simulink model "reservoir"  (R2016a)
settings: Solver=VariableStepAuto  StartTime=0.0  StopTime=10.0  RelTol=1e-3
settings Model: Creator=desilvtk  LastModifiedBy=desilvtk

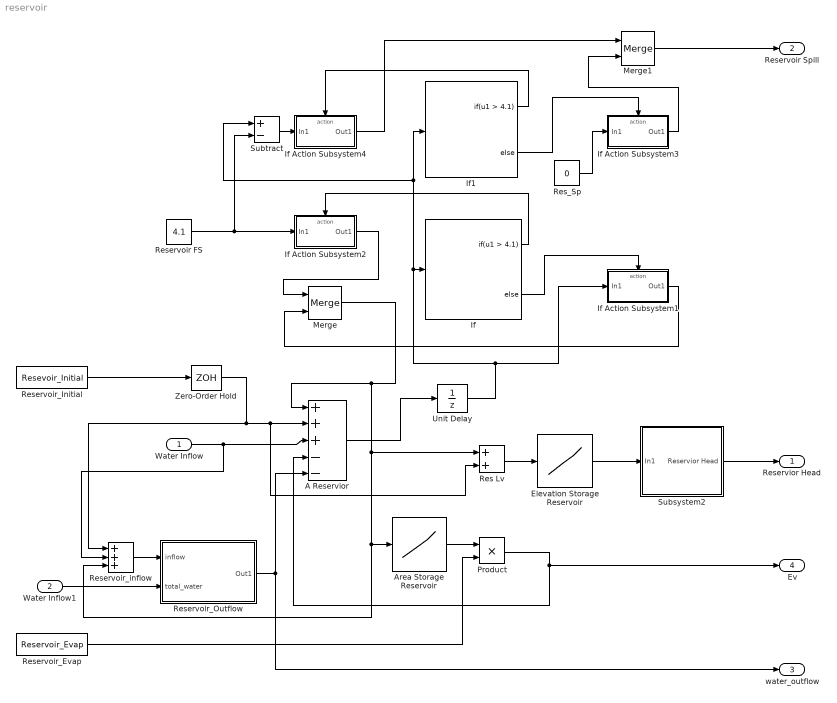
== system reservoir ==
  Water Inflow : Inport
  Water Inflow1 : Inport  Port=2
  A Reservior : Sum  Inputs=+++--
  Area Storage Reservoir : Lookup_n-D  NumberOfTableDimensions=1  BreakpointsForDimension1=[1.7,2.4,3.3,4.1]  UseOneInputPortForAllInputData=on  Table=[0.6,0.8,1,1.2]  InternalRulePriority=Speed  RndMeth=Simplest  InputSameDT=on
  Elevation Storage Reservoir : Lookup_n-D  NumberOfTableDimensions=1  BreakpointsForDimension1=[1.7,2.4,3.3,4.1]  UseOneInputPortForAllInputData=on  Table=[0,1,2,2]  InternalRulePriority=Speed  RndMeth=Simplest  InputSameDT=on
  If : If  IfExpression=u1 > 4.1
  If Action Subsystem1 : Subsystem  TreatAsAtomicUnit=on
  If Action Subsystem2 : Subsystem  TreatAsAtomicUnit=on
  If Action Subsystem3 : Subsystem  TreatAsAtomicUnit=on
  If Action Subsystem4 : Subsystem  TreatAsAtomicUnit=on
  If1 : If  IfExpression=u1 > 4.1
  Merge : Merge
  Merge1 : Merge
  Product : Product
  Res Lv : Sum
  Res_Sp : Constant  Value=0
  Reservoir FS : Constant  Value=4.1
  Reservoir_Evap : FromWorkspace  VariableName=Reservoir_Evap  SampleTime=0
  Reservoir_Initial : FromWorkspace  VariableName=Resevoir_Initial  SampleTime=0
  Reservoir_Outflow : Subsystem
  Reservoir_inflow : Sum  Inputs=+++
  Subsystem2 : Subsystem
  Subtract : Sum  Inputs=+-
  Unit Delay : UnitDelay
  Zero-Order Hold : ZeroOrderHold
  "Reservior Head " : Outport
  Reservoir Spill : Outport  Port=2
  water_outflow : Outport  Port=3
  Ev : Outport  Port=4
  wires:
  Zero-Order Hold/1 -> Res Lv/2, A Reservior/2, Reservoir_inflow/1
  If Action Subsystem1/1(Out1) -> Merge/2
  Merge/1 -> Res Lv/1, Area Storage Reservoir/1, Reservoir_inflow/3, A Reservior/1
  Reservoir_Initial/1 -> Zero-Order Hold/1
  Res Lv/1 -> Elevation Storage Reservoir/1
  A Reservior/1 -> Unit Delay/1
  Water Inflow/1 -> Reservoir_inflow/2, A Reservior/3
  If/2 -> If Action Subsystem1/Action
  Unit Delay/1 -> If Action Subsystem1/1(In1), Subtract/1, If1/1, If/1
  If Action Subsystem2/1(Out1) -> Merge/1
  Reservoir FS/1 -> Subtract/2, If Action Subsystem2/1(In1)
  If/1 -> If Action Subsystem2/Action
  If1/2 -> If Action Subsystem3/Action
  If1/1 -> If Action Subsystem4/Action
  Subtract/1 -> If Action Subsystem4/1(In1)
  Res_Sp/1 -> If Action Subsystem3/1(In1)
  If Action Subsystem4/1(Out1) -> Merge1/1
  If Action Subsystem3/1(Out1) -> Merge1/2
  Merge1/1 -> Reservoir Spill/1
  Area Storage Reservoir/1 -> Product/1
  Reservoir_inflow/1 -> Reservoir_Outflow/1(inflow)
  Reservoir_Outflow/1(Out1) -> water_outflow/1, A Reservior/5
  Elevation Storage Reservoir/1 -> Subsystem2/1(In1)
  Subsystem2/1("Reservior Head ") -> "Reservior Head "/1
  Product/1 -> Ev/1, A Reservior/4
  Reservoir_Evap/1 -> Product/2
  Water Inflow1/1 -> Reservoir_Outflow/2(total_water)

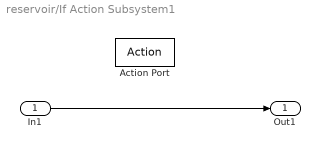
== system reservoir/If Action Subsystem1 ==
  In1 : Inport
  Action Port : ActionPort  ActionType=else
  Out1 : Outport
  wires:
  In1/1 -> Out1/1

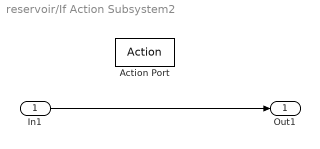
== system reservoir/If Action Subsystem2 ==
  In1 : Inport
  Action Port : ActionPort  ActionType=then
  Out1 : Outport
  wires:
  In1/1 -> Out1/1

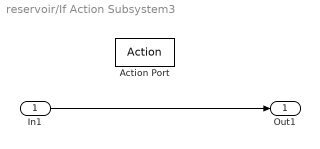
== system reservoir/If Action Subsystem3 ==
  In1 : Inport
  Action Port : ActionPort  ActionType=else
  Out1 : Outport
  wires:
  In1/1 -> Out1/1

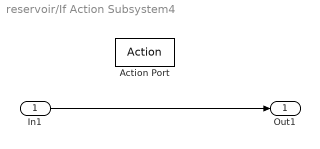
== system reservoir/If Action Subsystem4 ==
  In1 : Inport
  Action Port : ActionPort  ActionType=then
  Out1 : Outport
  wires:
  In1/1 -> Out1/1

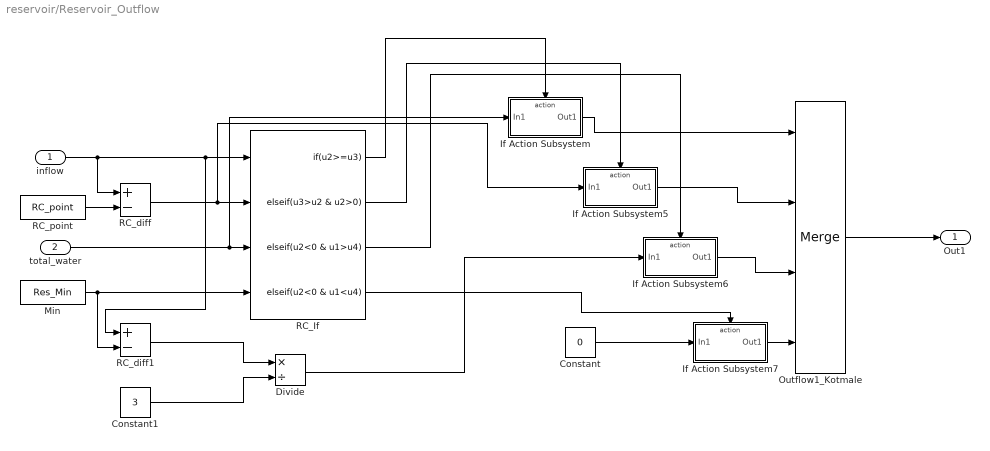
== system reservoir/Reservoir_Outflow ==
  inflow : Inport
  total_water : Inport  Port=2
  Constant : Constant  Value=0
  Constant1 : Constant  Value=3
  Divide : Product  Inputs=*/
  If Action Subsystem : Subsystem  TreatAsAtomicUnit=on
  If Action Subsystem5 : Subsystem  TreatAsAtomicUnit=on
  If Action Subsystem6 : Subsystem  TreatAsAtomicUnit=on
  If Action Subsystem7 : Subsystem  TreatAsAtomicUnit=on
  Min : FromWorkspace  VariableName=Res_Min  SampleTime=0
  Outflow1_Kotmale : Merge  Inputs=4
  RC_If : If  NumInputs=4  IfExpression=u2>=u3  ElseIfExpressions=u3>u2 & u2>0, u2<0 & u1>u4, u2<0 & u1<u4  ShowElse=off
  RC_diff : Sum  Inputs=+-
  RC_diff1 : Sum  Inputs=+-
  RC_point : FromWorkspace  VariableName=RC_point  SampleTime=0
  Out1 : Outport
  wires:
  RC_If/3 -> If Action Subsystem6/Action
  If Action Subsystem7/1(Out1) -> Outflow1_Kotmale/4
  inflow/1 -> RC_diff/1, RC_diff1/1, RC_If/1
  Outflow1_Kotmale/1 -> Out1/1
  total_water/1 -> RC_If/3, If Action Subsystem/1(In1)
  RC_diff/1 -> If Action Subsystem5/1(In1), RC_If/2
  RC_If/1 -> If Action Subsystem/Action
  If Action Subsystem6/1(Out1) -> Outflow1_Kotmale/3
  If Action Subsystem/1(Out1) -> Outflow1_Kotmale/1
  Constant/1 -> If Action Subsystem7/1(In1)
  RC_point/1 -> RC_diff/2
  If Action Subsystem5/1(Out1) -> Outflow1_Kotmale/2
  Min/1 -> RC_diff1/2, RC_If/4
  RC_If/2 -> If Action Subsystem5/Action
  RC_If/4 -> If Action Subsystem7/Action
  Constant1/1 -> Divide/2
  RC_diff1/1 -> Divide/1
  Divide/1 -> If Action Subsystem6/1(In1)

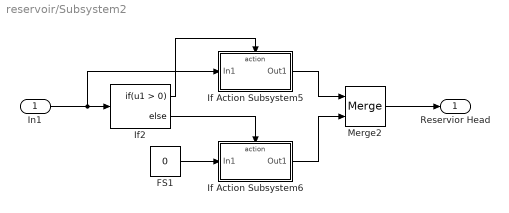
== system reservoir/Subsystem2 ==
  In1 : Inport
  " FS1" : Constant  Value=0
  If Action Subsystem5 : Subsystem  TreatAsAtomicUnit=on
  If Action Subsystem6 : Subsystem  TreatAsAtomicUnit=on
  If2 : If
  Merge2 : Merge
  "Reservior Head " : Outport
  wires:
  If Action Subsystem6/1(Out1) -> Merge2/2
  If Action Subsystem5/1(Out1) -> Merge2/1
  " FS1"/1 -> If Action Subsystem6/1(In1)
  In1/1 -> If Action Subsystem5/1(In1), If2/1
  If2/1 -> If Action Subsystem5/Action
  If2/2 -> If Action Subsystem6/Action
  Merge2/1 -> "Reservior Head "/1

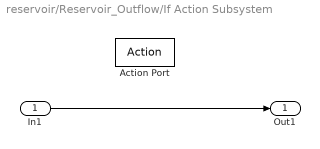
== system reservoir/Reservoir_Outflow/If Action Subsystem ==
  In1 : Inport
  Action Port : ActionPort
  Out1 : Outport
  wires:
  In1/1 -> Out1/1

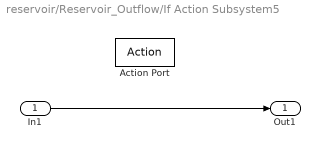
== system reservoir/Reservoir_Outflow/If Action Subsystem5 ==
  In1 : Inport
  Action Port : ActionPort
  Out1 : Outport
  wires:
  In1/1 -> Out1/1

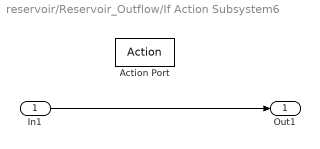
== system reservoir/Reservoir_Outflow/If Action Subsystem6 ==
  In1 : Inport
  Action Port : ActionPort
  Out1 : Outport
  wires:
  In1/1 -> Out1/1

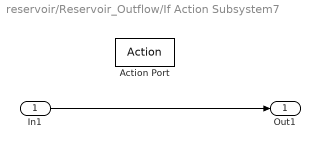
== system reservoir/Reservoir_Outflow/If Action Subsystem7 ==
  In1 : Inport
  Action Port : ActionPort
  Out1 : Outport
  wires:
  In1/1 -> Out1/1

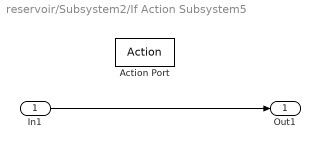
== system reservoir/Subsystem2/If Action Subsystem5 ==
  In1 : Inport
  Action Port : ActionPort
  Out1 : Outport
  wires:
  In1/1 -> Out1/1

== system reservoir/Subsystem2/If Action Subsystem6 ==
  In1 : Inport
  Action Port : ActionPort
  Out1 : Outport
  wires:
  In1/1 -> Out1/1
